simulink model "simu1"  (Simulink 7.4)
settings: Solver=ode45  StartTime=0.0  StopTime=5.0  RelTol=1e-3
settings Model: Creator=m134506  LastModifiedBy=m134506

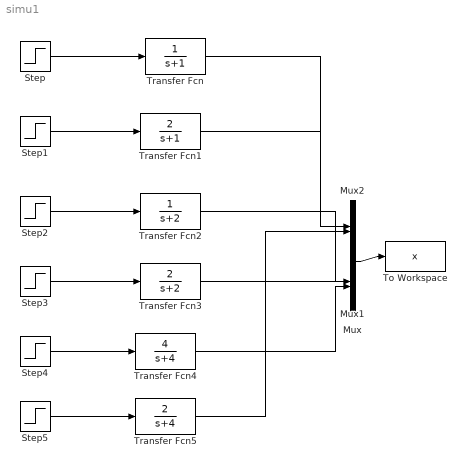
== system simu1 ==
  Mux : Mux  Inputs=2
  Mux1 : Mux  Inputs=2
  Mux2 : Mux  Inputs=2
  Step{,1..5} (6 alike) : Step  Time=0  SampleTime=0
  To Workspace : ToWorkspace  VariableName=x  SampleTime=-1  SaveFormat=Array
  Transfer Fcn : TransferFcn  Denominator=[1 1]
  Transfer Fcn1 : TransferFcn  Numerator=[2]  Denominator=[1 1]
  Transfer Fcn2 : TransferFcn  Denominator=[1 2]
  Transfer Fcn3 : TransferFcn  Numerator=2  Denominator=[1 2]
  Transfer Fcn4 : TransferFcn  Numerator=4  Denominator=[1 4]
  Transfer Fcn5 : TransferFcn  Numerator=2  Denominator=[1 4]
  wires:
  Step/1 -> Transfer Fcn/1
  Step1/1 -> Transfer Fcn1/1
  Step2/1 -> Transfer Fcn2/1
  Step3/1 -> Transfer Fcn3/1
  Step4/1 -> Transfer Fcn4/1
  Step5/1 -> Transfer Fcn5/1
  Transfer Fcn5/1 -> Mux/1
  Transfer Fcn4/1 -> Mux/2
  Transfer Fcn3/1 -> Mux1/2
  Transfer Fcn2/1 -> Mux1/1
  Transfer Fcn1/1 -> Mux2/1
  Transfer Fcn/1 -> Mux2/2
  Mux/1 -> To Workspace/1
